simulink model "SinglePhaseFullwaveSemiControlled"  (R2025a)
settings: Solver=VariableStepAuto  StartTime=0.0  StopTime=0.1  RelTol=1e-3
values from neighbouring files (symbols this model uses):
  A = zeros(Rows,nbus)    [EXP 3_Y_BUS_BY_SINGULAR_TRANSFORMATION.m]    (also in T-MODEL.m = 1 + (Y * Z)/2; code2.m = 1 + (Y * Z)/2; code3.m = 1 + (Y * Z)/2; code4.m = cosh(gamma*l))
libraries: spsDiodeLib x2, spsThyristorLib x2, spsVoltageMeasurementLib x2, spsACVoltageSourceLib x1, spsDCVoltageSourceLib x1, spsDCMachineLib x1, sps_lib x1
settings Model: Creator=HP  LastModifiedBy=samar

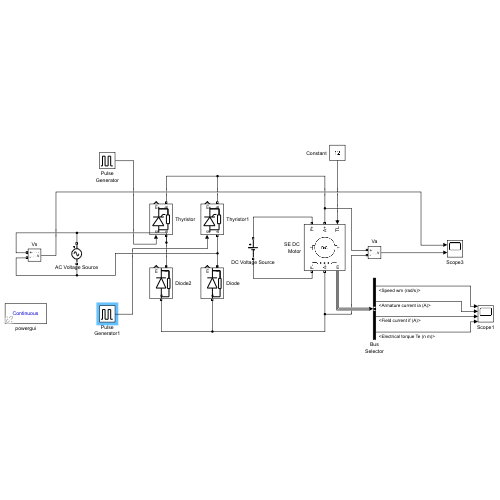
[thumbnail: Simulink's stored preview of the top-level diagram]
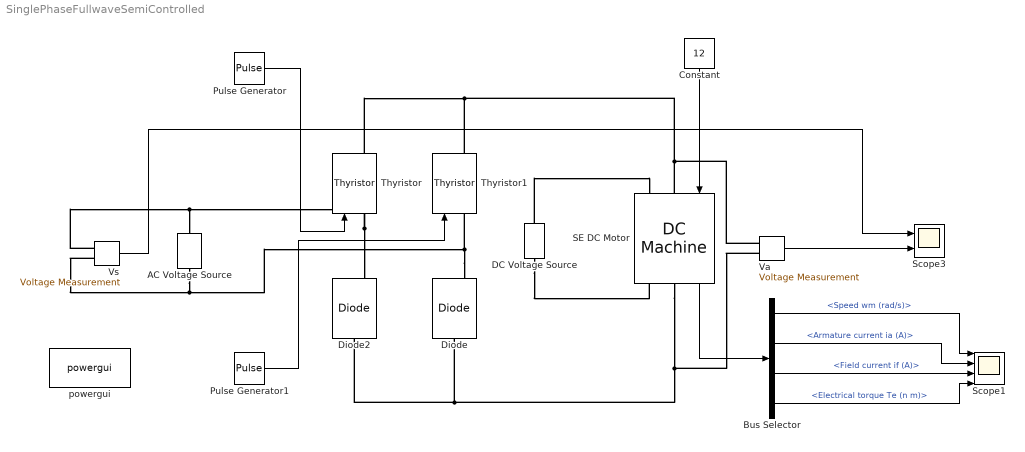
== system SinglePhaseFullwaveSemiControlled ==
  AC Voltage Source : spsACVoltageSourceLib/AC Voltage Source  Amplitude=220  Phase=0  Frequency=50  SampleTime=0  Measurements=None  BusType=swing  Pref=10e3  Qref=0  Qmin=-inf  Qmax=+inf
  Bus Selector : BusSelector  OutputSignals=Speed wm (rad/s),Armature current ia (A),Field current if (A),Electrical torque Te (n m)
  Constant : Constant  Value=12
  DC Voltage Source : spsDCVoltageSourceLib/DC Voltage Source  Amplitude=200  Measurements=None
  Diode : spsDiodeLib/Diode  Ron=0.001  Lon=0  Vf=0.8  IC=0  UseSnubber=0  Rs=500  Cs=250e-9  Measurements=on
  Diode2 : spsDiodeLib/Diode  Ron=0.001  Lon=0  Vf=0.8  IC=0  UseSnubber=0  Rs=500  Cs=250e-9  Measurements=on
  Pulse Generator : DiscretePulseGenerator  PulseType=Time based  Amplitude=5  Period=1/50  PulseWidth=5  PhaseDelay=(30/360)*0.02
  Pulse Generator1 : DiscretePulseGenerator  PulseType=Time based  Amplitude=5  Period=1/50  PulseWidth=5  PhaseDelay=(210/360)*0.02
  SE DC Motor : spsDCMachineLib/DC Machine  PresetModel=No  MechanicalLoad=Torque TL  FieldType=Wound  ShowDetailedParameters=on  MeasurementBus=off  RLa="[ 0.6  0.2]"  RLf="[ 240  120]"  Laf=1.8  MachineConstant=Torque constant (N.m/A)  Ke=1.8  Kt=1.8  J=1  Bm=0  Tf=0  w0=1  Ifinit=0.833333332510866  TsPowergui=0  TsBlock=-1
  Scope1 : Scope  NumInputPorts=4
      settings: ActiveDisplayYMinimum=0.52196444681309073  ActiveDisplayYMaximum=4.4806971221211063
  Scope3 : Scope  NumInputPorts=2
      settings: ActiveDisplayYMinimum=-279.84992829527789  ActiveDisplayYMaximum=297.56178396381131  DataLoggingVariableName=ScopeData3
  Thyristor : spsThyristorLib/Thyristor  Ron=0.001  Lon=0  Vf=0.8  IC=0  Rs=500  Cs=250e-9  Measurements=on
  Thyristor1 : spsThyristorLib/Thyristor  Ron=0.001  Lon=0  Vf=0.8  IC=0  Rs=500  Cs=250e-9  Measurements=on
  Va : spsVoltageMeasurementLib/Voltage Measurement  PhasorSimulation=off  OutputType=Complex  PSBequivalent=0
  Vs : spsVoltageMeasurementLib/Voltage Measurement  PhasorSimulation=off  OutputType=Complex  PSBequivalent=0
  powergui : sps_lib/powergui  Priority=1  SimulationMode=Continuous  SampleTime=50e-6  frequency=60  Iterations=50  frequencyindice=50  Pbase=100e6  ErrMax=1e-4  UnitsV=kV  UnitsW=MW  buscounter=0  FunctionMessages=off  echomessages=off  EnableUseOfTLC=off  CurrentSourceSwitches=off  DisableSnubberDevices=off  DisableRonSwitches=off  DisableVfSwitches=off  DisplayEquations=off  AutomaticDiscreteSolvers=off  SolverType=Tustin/Backward Euler (TBE)  Interpol=off  ExternalGateDelay=off  methode=off  Ts=100  x0status=blocks  SPID=on  SwTol=0  HookPort=off  NonlinearTolerance=1e-4  nMaxIteration=100  ContinueOnMaxIteration=off  RestoreLinks=warning  ResistiveCurrentMeasurement=off  Frange=[0:2:500]  Ylog=off  Xlog=on  ShowGrid=off  save=off  variable=ZData  structure=0  ZoomFFT=off  StartTime=0.0  cycles=1  DisplayStyle=1  fundamental=60  FreqAxis=off  MaxFrequency=1000  frequencyindicesteady=1  RmsSteady=1  display=off
  wires:
  Pulse Generator1/1 -> Thyristor1/1
  Constant/1 -> SE DC Motor/1
  Pulse Generator/1 -> Thyristor/1
  Bus Selector/3 -> Scope1/3  "<Field current if (A)>"
  Bus Selector/2 -> Scope1/2  "<Armature current ia (A)>"
  SE DC Motor/1 -> Bus Selector/1
  Bus Selector/4 -> Scope1/4  "<Electrical torque Te (n m)>"
  Bus Selector/1 -> Scope1/1  "<Speed wm (rad/s)>"
  Vs/1 -> Scope3/1
  Va/1 -> Scope3/2
  connections:
  Vs/LConn1 -- AC Voltage Source/RConn1 -- Diode2/RConn1 -- Thyristor/LConn1
  Va/LConn1 -- Thyristor/RConn1 -- Thyristor1/RConn1 -- SE DC Motor/LConn1
  Diode/RConn1 -- Thyristor1/LConn1 -- AC Voltage Source/LConn1 -- Vs/LConn2
  Va/LConn2 -- SE DC Motor/RConn1 -- Diode2/LConn1 -- Diode/LConn1
  DC Voltage Source/RConn1 -- SE DC Motor/LConn2
  DC Voltage Source/LConn1 -- SE DC Motor/RConn2
